simulink model "turret_system"  (R2025b)
settings: Solver=VariableStepAuto  StartTime=0.0  StopTime=10.0  RelTol=1e-3
values from neighbouring files (symbols this model uses):
  dt_ms = 0.001    [motor_characterization.m]    (also in pid_autotuning.m = 15)
  lead_den = [1, 1]    [motor_characterization.m]
  lead_num = [3.819, 1]    [motor_characterization.m]
undefined symbols (not defined in the file or in its folder): a, b
libraries: slpidlib x1
settings Model: Creator=Arihant  LastModifiedBy=Arihant

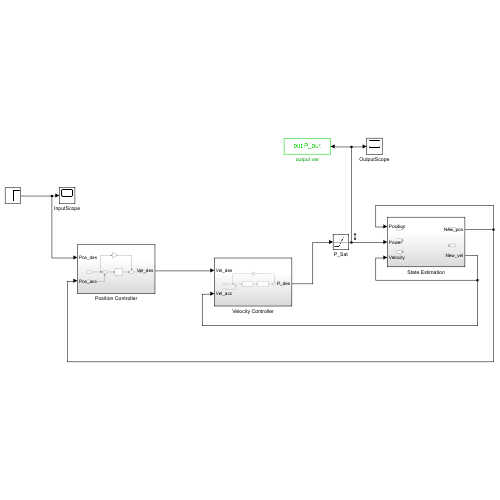
[thumbnail: Simulink's stored preview of the top-level diagram]
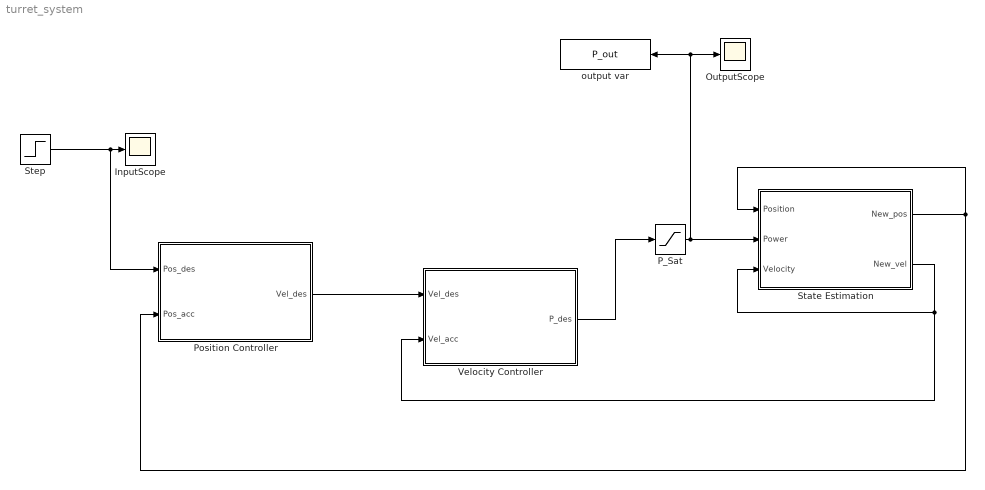
== system turret_system ==
  InputScope : Scope
  OutputScope : Scope
  P_Sat : Saturate  UpperLimit=16000  LowerLimit=-16000
  Position Controller : Subsystem
  State Estimation : Subsystem
  Step : Step  Time=.05  After=170  SampleTime=0
  Velocity Controller : Subsystem
  output var : ToWorkspace  VariableName=P_out  SampleTime=-1
      settings: Save2DSignal=2-D array (concatenate along first dimension)
  wires:
  P_Sat/1 -> output var/1, OutputScope/1, State Estimation/2(Power)
  State Estimation/2(New_vel) -> State Estimation/3(Velocity), Velocity Controller/2(Vel_acc)
  Position Controller/1(Vel_des) -> Velocity Controller/1(Vel_des)
  Velocity Controller/1(P_des) -> P_Sat/1
  State Estimation/1(New_pos) -> State Estimation/1(Position), Position Controller/2(Pos_acc)
  Step/1 -> Position Controller/1(Pos_des), InputScope/1

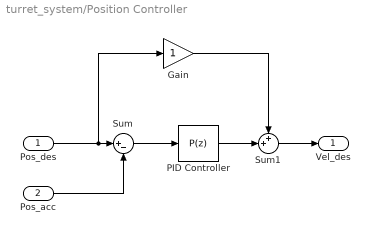
== system turret_system/Position Controller ==
  Pos_des : Inport
  Pos_acc : Inport  Port=2
  Gain : Gain
  PID Controller : slpidlib/PID Controller  Controller=P  Form=Parallel  TimeDomain=Discrete-time  UseExternalTs=off  SampleTime=dt_ms  IntegratorMethod=Forward Euler  FilterMethod=Forward Euler  ControllerParametersSource=internal  P=1  I=1  UseKiTs=off  D=0  UseExternalDerivativeSource=off  N=100  UseFilter=on  TunerSelectOption=Transfer Function Based (PID Tuner App)  InitialConditionSource=internal  InitialConditionForIntegrator=0  InitialConditionForFilter=0  DifferentiatorICPrevScaledInput=0  ExternalReset=none  TrackingMode=off  Kt=1  LimitOutput=off  SatLimitsSource=internal  UpperSaturationLimit=inf  LowerSaturationLimit=-inf  LinearizeAsGain=on  AntiWindupMode=none  Kb=1  LimitIntegrator=off  UpperIntegratorSaturationLimit=inf  LowerIntegratorSaturationLimit=-inf  POutMin=[]  POutMax=[]  IOutMin=[]  IOutMax=[]  DOutMin=[]  DOutMax=[]  NOutMin=[]  NOutMax=[]  SumOutMin=[]  SumOutMax=[]  SaturationOutMin=[]  SaturationOutMax=[]  PParamMin=[]  PParamMax=[]  IParamMin=[]  IParamMax=[]  DParamMin=[]  DParamMax=[]  NParamMin=[]  NParamMax=[]  KbParamMin=[]  KbParamMax=[]  KtParamMin=[]  KtParamMax=[]  KbOutMin=[]  KbOutMax=[]  KtOutMin=[]  KtOutMax=[]  IntegratorOutMin=[]  IntegratorOutMax=[]  FilterOutMin=[]  FilterOutMax=[]  SumI1OutMin=[]  SumI1OutMax=[]  SumI2OutMin=[]  SumI2OutMax=[]  SumI3OutMin=[]  SumI3OutMax=[]  SumI4OutMin=[]  SumI4OutMax=[]  SumDOutMin=[]  SumDOutMax=[]  DifferentiatorOutMin=[]  DifferentiatorOutMax=[]  FilterDiffOutCoefMin=[]  FilterDiffOutCoefMax=[]  ReciprocalOutMin=[]  ReciprocalOutMax=[]  SumDenOutMin=[]  SumDenOutMax=[]  SumNumOutMin=[]  SumNumOutMax=[]  DivideOutMin=[]  DivideOutMax=[]  UdiffTsProdOutMin=[]  UdiffTsProdOutMax=[]  NTsProdOutMin=[]  NTsProdOutMax=[]  UintegralTsProdOutMin=[]  UintegralTsProdOutMax=[]  UngainTsProdOutMin=[]  UngainTsProdOutMax=[]  ClampingZeroOutDataTypeStr=Inherit: Inherit via back propagation  ClampingZeroOutMin=[]  ClampingZeroOutMax=[]  FilterDenConstantOutDataTypeStr=Inherit: Inherit via back propagation  FilterDenConstantOutMin=[]  FilterDenConstantOutMax=[]  PCopyOutDataTypeStr=Inherit: Inherit via back propagation  PCopyOutMin=[]  PCopyOutMax=[]  NCopyOutDataTypeStr=Inherit: Inherit via back propagation  NCopyOutMin=[]  NCopyOutMax=[]  IntegratorContinuousStateAttributes=''  IntegratorStateMustResolveToSignalObject=off  IntegratorRTWStateStorageClass=Auto  FilterContinuousStateAttributes=''  FilterStateMustResolveToSignalObject=off  FilterRTWStateStorageClass=Auto  ParallelPVariant=InternalParameters  IdealPVariant=Disabled  IVariant=Disabled  DVariant=Disabled  IntegratorVariant=Disabled  SatVariant=Disabled  AWVariant=Disabled  PCopyVariant=Disabled  TRVariant=Disabled  FdbkBlocksVariant=Forward  IdealPFdbkVariant=Disabled  SatFdbkVariant=Disabled  DerivativeFilterVariant=Disabled  NVariant=Disabled  NCopyVariant=Disabled_SignalSpec  FilterICVariant=Disabled  IntegratorICVariant=Disabled  ExternalResetVariant=Disabled  TRSumVariant=Passthrough  SumFdbkVariant=Disabled  SumVariant=Passthrough_P  TsampFilterVariant=InternalTs  TsampNgainVariant=Passthrough  TsampIntegralVariant=Disabled_SignalSpec  ExternalSaturationOutDataTypeStr=Inherit: Same as second input  DerivativeSourceVariant=Disabled  PreIntVariant=InternalPreInt
  Sum : Sum  Inputs=|+-
  Sum1 : Sum  Inputs=++|
  Vel_des : Outport
  wires:
  Pos_des/1 -> Gain/1, Sum/1
  Pos_acc/1 -> Sum/2
  Sum/1 -> PID Controller/1
  Gain/1 -> Sum1/1
  PID Controller/1 -> Sum1/2
  Sum1/1 -> Vel_des/1

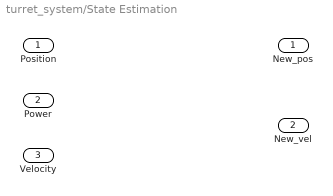
== system turret_system/State Estimation ==
  Position : Inport
  Power : Inport  Port=2
  Velocity : Inport  Port=3
  New_pos : Outport
  New_vel : Outport  Port=2

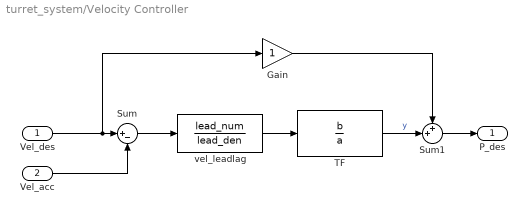
== system turret_system/Velocity Controller ==
  Vel_des : Inport
  Vel_acc : Inport  Port=2
  Gain : Gain
  Sum : Sum  Inputs=|+-
  Sum1 : Sum  Inputs=++|
  TF : TransferFcn  Numerator=b  Denominator=a  ContinuousStateAttributes='velocity'
  vel_leadlag : TransferFcn  Numerator=lead_num  Denominator=lead_den  ContinuousStateAttributes='velocity'
  P_des : Outport
  wires:
  vel_leadlag/1 -> TF/1
  Vel_des/1 -> Gain/1, Sum/1
  Vel_acc/1 -> Sum/2
  Sum/1 -> vel_leadlag/1
  Gain/1 -> Sum1/1
  TF/1 -> Sum1/2  "y"
  Sum1/1 -> P_des/1
